simulink model "LOAD_UNIT_TEST"  (Simulink 7.8)
settings: Solver=ode1  StartTime=0.0  StopTime=60  FixedStep=Ts  MaxStep=1e-3  RelTol=1e-3
model workspace (MAT data in the model file):
  op_snapshot1 : opcond.OperatingPoint (value not decoded)
PostLoadFcn:
  | Ts=80e-6;
InitFcn:
  | Ts=80e-6;
libraries: powerlib x5, cables_lib x3, modbus_lib x3, dynamic_load_lib x2, transformer_lib x1, artemis x1, rtlab x1
settings Model: ARTEMISmethode_block_infos=$$__separator__$$LOAD_UNIT_TEST/ARTEMIS Guide$$__separator__$$  Creator=RE25624  LastModifiedBy=RE25624  BufferReuse=off
settings SolverCC: ZeroCrossAlgorithm=Adaptive
settings DataIOCC: ExternalInput=getinputstruct(op_snapshot1)  InitialState=getstatestruct(op_snapshot1)  LimitDataPoints=off  MaxDataPoints=90060  SignalLoggingSaveFormat=Dataset  SaveOutput=off  SignalLogging=off  DSMLogging=off  SaveTime=off  OutputSaveName=result
settings OptimizationCC: BlockReduction=off  OptimizeBlockIOStorage=off  BufferReuse=off  ExpressionFolding=off  LocalBlockOutputs=off
settings DebuggingCC: MaxConsecutiveZCsMsg=warning  IgnoredZcDiagnostic=none  SolverPrmCheckMsg=none  MultiTaskRateTransMsg=warning  FrameProcessingCompatibilityMsg=error  ModelReferenceExtraNoncontSigs=warning  StrictBusMsg=None
settings ModelReferenceCC: UpdateModelReferenceTargets=IfOutOfDate
settings SFSimCC: SFSimEcho=off
settings GRTTargetCC: TargetFunctionLibrary=C89/C90 (ANSI)

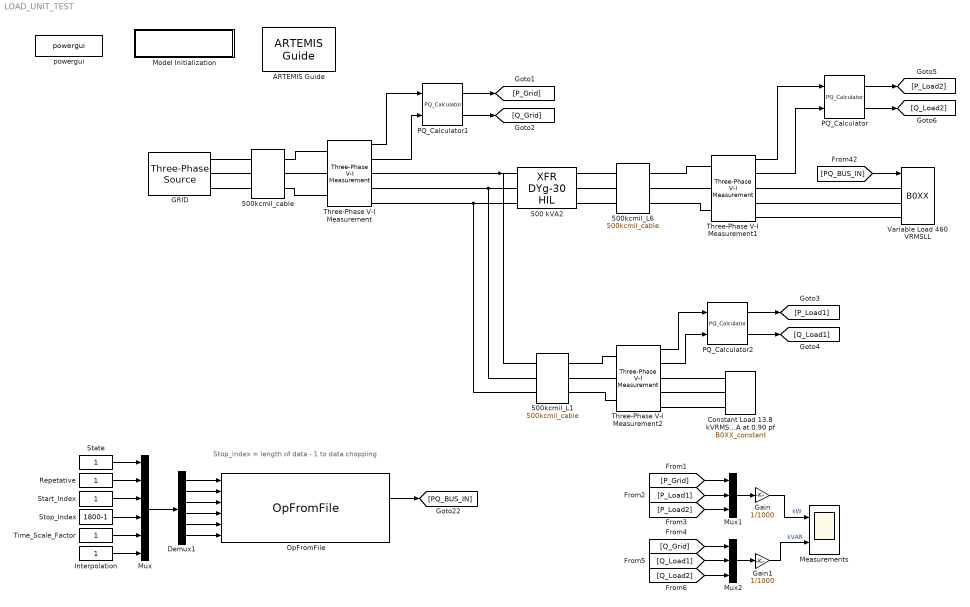
== system LOAD_UNIT_TEST ==
  note: Stop_index = length of data - 1 to data chopping
  500 kVA2 : transformer_lib/XFR DYg-30 HIL  Rating=500  Vp=13800  Vs=460  Z=5  XR=4.9
  500kcmil_L1 : cables_lib/500kcmil_cable  length=300  par_sets=1
  500kcmil_L6 : cables_lib/500kcmil_cable  length=50  par_sets=1
  500kcmil_cable : cables_lib/500kcmil_cable  length=1000  par_sets=1
  ARTEMIS Guide : artemis/ARTEMIS/ARTEMIS Guide  Tag=FTSSmethode_opal_4hx0r99  Description=5.0_z1  lock=on  Ts=Ts  opt=art5  dyna=off  nb_perm=4  RT_fullcomp=off  ssn=on  ssn_itvc=off  ssn_ivic=off  ssn_ext=off  ssn_solver=Art5 with Backward Euler nodal interface  ssn_impulse=off  ssn_quasimpulse=off  ssn_impulse_loop=2  paraExtinctionThy=off  Thy_Impulse=on  dtc=Off  dtc_opt=normal  ao=on  simtype=off  ct_mac=off  lin_mov=off  lsp=[0.001 2]  spike_skip=Disabled  dtc_extra=1  dtc_sws=normal  dtc_pied=0.5  SPSRulesBlock=SPSRules  tre=on  ctmm=off  LF=off  dpl_type=ARTEMiS DPL  rlc_type=off  custom_type=off  para=on  ssn_ImpulseLoopBlockedStateUpdate=2  ssn_mov_iter_number=5  ssn_switch_iter_number=5
  Constant Load 13.8 kVRMSLL 5000 kVA at 0.90 pf : dynamic_load_lib/B0XX_constant  v=13800  kVA=5000  pf=0.90
  Demux1 : Demux  Outputs=6
  GRID : powerlib/Electrical Sources/Three-Phase Source  Voltage=13800  PhaseAngle=0  Frequency=60  InternalConnection=Yg  SpecifyImpedance=on  Resistance=0.8929  Inductance=16.58e-3  ShortCircuitLevel=375e6  BaseVoltage=13800  XRratio=7.9  BusType=swing  Pref=0  Qref=0  Qmin=-inf  Qmax=inf
  Gain : Gain  Gain=1/1000
  Gain1 : Gain  Gain=1/1000
  "Interpolation " : Constant
  Measurements : Scope  NumInputPorts=2
      settings: TimeRange=60  YMin=-1000~-500  YMax=7000~3500
  Model Initialization : Subsystem  AncestorBlock=artemis/Tools /Misc/Model Initialization  mask(Model Functions){InitFcnX=Ts=80e-6;, prel=off, posl=on, inif=on, strf=off}
      mask prompts: InitFcnX "Initialisation"; prel "Preload Function"; posl "PostLoad Function"; inif "InitFcn"; strf "StartFcn"
      mask init:
      | currentBlock = gcb;
      | root = bdroot(currentBlock);
      | 
      | if ~strcmp(get_param(root,'BlockDiagramType'),'library')
      |     if prel==1
      |         set_param(root, 'PreLoadFcn', InitFcnX);
      |     else
      |         set_param(root, 'PreLoadFcn', '');
      |     end
      |     if inif==1
      |         set_param(root, 'InitFcn', InitFcnX);
      |     else
      |         set_param(root, 'InitFcn', '');
      |     end
      |     if strf==1
      |         set_param(root, 'StartFcn', InitFcnX);
      |     else
      |         set_param(root, 'StartFcn', '');
      |     end
      |     if posl==1
      |         set_param(root, 'PostLoadFcn', InitFcnX);
      |     else
      |         set_param(root, 'PostLoadFcn', '');
      |     end
      | end
      | 
      | pos = get_param(currentBlock, 'Position');
      | width = pos(3) - pos(1); height = pos(4) - pos(2);
      | txt = [ upper(root) '\n' '- InitFcn. . . . . '  get_param(root, 'InitFcn') ];
      settings: CopyFcn=set_param(gcb,'LinkStatus','inactive')
      mask Display: text(5, height*0.5, txt, 'horizontalAlignment', 'left', 'verticalAlignment', 'middle') ;
  Mux : Mux  Inputs=6
  Mux1 : Mux  Inputs=3
  Mux2 : Mux  Inputs=3
  OpFromFile : rtlab/DataLogging/OpFromFile  filename_mode=Static (same filename all the time)  reload_mode=Next time model is paused (Real-Time)  init_file_id=0  filename=one_min_data.mat  rtpath='./'  nrtpath='.\'  sample_time=0
  PQ_Calculator : modbus_lib/SEL_787_Relay/PQ_Calculator
  PQ_Calculator1 : modbus_lib/SEL_787_Relay/PQ_Calculator
  PQ_Calculator2 : modbus_lib/SEL_787_Relay/PQ_Calculator
  "Repetative " : Constant
  "Start_Index " : Constant
  "State " : Constant
  "Stop_Index " : Constant  Value=1800-1
  Three-Phase V-I Measurement : powerlib/Measurements/Three-Phase V-I Measurement  VoltageMeasurement=phase-to-ground  SetLabelV=off  LabelV=Vabc  Vpu=off  VpuLL=off  CurrentMeasurement=yes  SetLabelI=off  LabelI=Iabc  Ipu=off  Pbase=100e6  Vbase=500e3  OutputType=Complex  PhasorSimulation=off  PSBequivalent=0
  Three-Phase V-I Measurement1 : powerlib/Measurements/Three-Phase V-I Measurement  VoltageMeasurement=phase-to-ground  SetLabelV=off  LabelV=Vabc  Vpu=off  VpuLL=off  CurrentMeasurement=yes  SetLabelI=off  LabelI=Iabc  Ipu=off  Pbase=100e6  Vbase=500e3  OutputType=Complex  PhasorSimulation=off  PSBequivalent=0
  Three-Phase V-I Measurement2 : powerlib/Measurements/Three-Phase V-I Measurement  VoltageMeasurement=phase-to-ground  SetLabelV=off  LabelV=Vabc  Vpu=off  VpuLL=off  CurrentMeasurement=yes  SetLabelI=off  LabelI=Iabc  Ipu=off  Pbase=100e6  Vbase=500e3  OutputType=Complex  PhasorSimulation=off  PSBequivalent=0
  "Time_Scale_Factor " : Constant
  Variable Load 460 VRMSLL : dynamic_load_lib/B0XX  V=460  P_Scale=2  Q_Scale=2
  powergui : powerlib/powergui  Priority=2  SimulationMode=Discrete  SolverType=Tustin  SampleTime=Ts  frequency=60  SPID=off  DisableSnubberDevices=off  DisableRonSwitches=off  DisableVfSwitches=off  SwTol=0  Interpol=off  DisplayEquations=off  FunctionMessages=off  frequencyindice=0  Pbase=100e6  ErrMax=1e-4  Iterations=50  UnitsV=kV  UnitsW=MW  echomessages=off  HookPort=off  EnableUseOfTLC=off  x0status=blocks  RestoreLinks=warning  ResistiveCurrentMeasurement=off  Frange=logspace(0,3,50)  Ylog=off  Xlog=off  ShowGrid=off  save=off  variable=ZData  structure=0  ZoomFFT=on  StartTime=0.0  cycles=2  DisplayStyle=off  fundamental=60  FreqAxis=off  MaxFrequency=1000  frequencyindicesteady=1  RmsSteady=1  display=off  Ts=0  methode=off
  wires:
  [PQ_BUS_IN] -> Variable Load 460 VRMSLL/1
  Demux1/6 -> OpFromFile/6
  Demux1/5 -> OpFromFile/5
  Demux1/4 -> OpFromFile/4
  Demux1/3 -> OpFromFile/3
  Demux1/2 -> OpFromFile/2
  Demux1/1 -> OpFromFile/1
  Mux/1 -> Demux1/1
  "Interpolation "/1 -> Mux/6
  "Time_Scale_Factor "/1 -> Mux/5
  "Stop_Index "/1 -> Mux/4
  "Start_Index "/1 -> Mux/3
  "Repetative "/1 -> Mux/2
  "State "/1 -> Mux/1
  Three-Phase V-I Measurement1/1 -> PQ_Calculator/1
  Three-Phase V-I Measurement1/2 -> PQ_Calculator/2
  Three-Phase V-I Measurement/1 -> PQ_Calculator1/1
  Three-Phase V-I Measurement/2 -> PQ_Calculator1/2
  OpFromFile/2 -> [PQ_BUS_IN]
  Three-Phase V-I Measurement2/1 -> PQ_Calculator2/1
  Three-Phase V-I Measurement2/2 -> PQ_Calculator2/2
  Mux2/1 -> Gain1/1
  Mux1/1 -> Gain/1
  PQ_Calculator1/1 -> [P_Grid]
  PQ_Calculator1/2 -> [Q_Grid]
  PQ_Calculator/1 -> [P_Load2]
  PQ_Calculator/2 -> [Q_Load2]
  PQ_Calculator2/1 -> [P_Load1]
  PQ_Calculator2/2 -> [Q_Load1]
  [P_Grid] -> Mux1/1
  [P_Load1] -> Mux1/2
  [P_Load2] -> Mux1/3
  [Q_Grid] -> Mux2/1
  [Q_Load1] -> Mux2/2
  [Q_Load2] -> Mux2/3
  Gain/1 -> Measurements/1  "kW"
  Gain1/1 -> Measurements/2  "kVAR"
  connections:
  500kcmil_cable/LConn1 -- GRID/RConn1
  Three-Phase V-I Measurement/LConn2 -- 500kcmil_cable/RConn2
  500kcmil_cable/LConn2 -- GRID/RConn2
  Three-Phase V-I Measurement/LConn1 -- 500kcmil_cable/RConn1
  500kcmil_cable/LConn3 -- GRID/RConn3
  Three-Phase V-I Measurement/LConn3 -- 500kcmil_cable/RConn3
  500kcmil_L6/LConn3 -- 500 kVA2/RConn3
  500kcmil_L6/LConn2 -- 500 kVA2/RConn2
  500kcmil_L6/LConn1 -- 500 kVA2/RConn1
  500 kVA2/LConn3 -- Three-Phase V-I Measurement/RConn3 -- 500kcmil_L1/LConn3
  Three-Phase V-I Measurement/RConn2 -- 500 kVA2/LConn2 -- 500kcmil_L1/LConn2
  Three-Phase V-I Measurement/RConn1 -- 500 kVA2/LConn1 -- 500kcmil_L1/LConn1
  Three-Phase V-I Measurement1/LConn3 -- 500kcmil_L6/RConn3
  Three-Phase V-I Measurement1/LConn2 -- 500kcmil_L6/RConn2
  Three-Phase V-I Measurement1/LConn1 -- 500kcmil_L6/RConn1
  Variable Load 460 VRMSLL/LConn3 -- Three-Phase V-I Measurement1/RConn3
  Variable Load 460 VRMSLL/LConn2 -- Three-Phase V-I Measurement1/RConn2
  Variable Load 460 VRMSLL/LConn1 -- Three-Phase V-I Measurement1/RConn1
  Three-Phase V-I Measurement2/RConn3 -- Constant Load 13.8 kVRMSLL 5000 kVA at 0.90 pf/LConn3
  Three-Phase V-I Measurement2/RConn2 -- Constant Load 13.8 kVRMSLL 5000 kVA at 0.90 pf/LConn2
  Three-Phase V-I Measurement2/RConn1 -- Constant Load 13.8 kVRMSLL 5000 kVA at 0.90 pf/LConn1
  Three-Phase V-I Measurement2/LConn3 -- 500kcmil_L1/RConn3
  Three-Phase V-I Measurement2/LConn2 -- 500kcmil_L1/RConn2
  Three-Phase V-I Measurement2/LConn1 -- 500kcmil_L1/RConn1

== system LOAD_UNIT_TEST/Model Initialization ==
